simulink model "test_dram_vacc_out"  (Simulink 6.2)
settings: Solver=ode45  StartTime=0.0  StopTime=30000  RelTol=1e-3
undefined symbols (not defined in the file): ant_bits, blockCountBits, blockRowBits
libraries: xbsIndex_r3 x678, xps_library x31, casper_library x10
(part 1 of 4)
settings Model: LastModifiedBy=Jason Manley
settings DebuggingCC: SolverPrmCheckMsg=warning

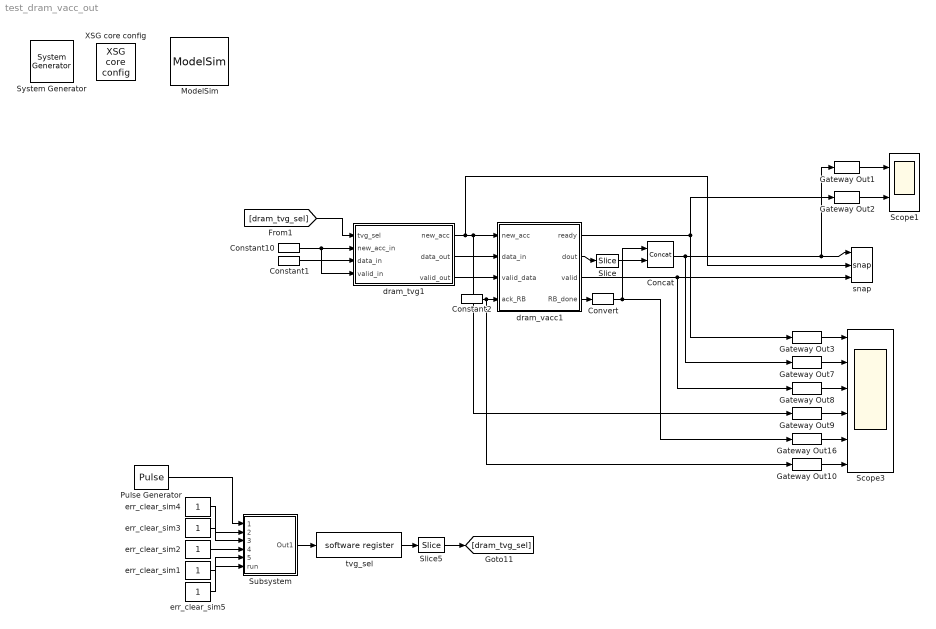
== system test_dram_vacc_out ==
  " System Generator" : xbsIndex_r3/ System Generator  Tag=genX  xilinxfamily=Virtex2P  part=xc2vp70  speed=-7  package=ff1704  synthesis_tool=XST  directory=./dram_acc_test8/sysgen  testbench=off  simulink_period=1  sysclk_period=4.878  incr_netlist=off  trim_vbits=Everywhere in SubSystem  dbl_ovrd=According to Block Masks  core_generation=According to Block Masks  run_coregen=off  deprecated_control=off  eval_field=0
      settings: AttributesFormatString=System\nGenerator
  Concat : xbsIndex_r3/Concat  num_inputs=2  explicit_period=off  period=1  dbl_ovrd=off
  Constant1 : xbsIndex_r3/Constant  const=0  equ=P=C  arith_type=Unsigned  n_bits=128  bin_pt=0  opselect=C  inp2=PCIN>>17  opr=+  inp1=P  carry=CIN  iostate=0  explicit_period=on  period=1  dbl_ovrd=off
  Constant10 : xbsIndex_r3/Constant  const=0  equ=P=C  arith_type=Boolean  n_bits=1  bin_pt=0  opselect=C  inp2=PCIN>>17  opr=+  inp1=P  carry=CIN  iostate=0  explicit_period=on  period=1  dbl_ovrd=off
  Constant2 : xbsIndex_r3/Constant  const=1  equ=P=C  arith_type=Boolean  n_bits=1  bin_pt=0  opselect=C  inp2=PCIN>>17  opr=+  inp1=P  carry=CIN  iostate=0  explicit_period=on  period=1  dbl_ovrd=off
  Convert : xbsIndex_r3/Convert  arith_type=Unsigned  n_bits=1  bin_pt=0  quantization=Truncate  overflow=Wrap  latency=0  explicit_period=off  period=1  dbl_ovrd=off  show_param=off  inserted_by_tool=off  pipeline=off
      settings: xl_area=[0, 0, 0, 0, 0, 0, 0]
  Gateway Out{1..3,7..10,16} (8 alike) : xbsIndex_r3/Gateway Out  output_type=Double  nbits=8  bin_pt=6  arith_type=Boolean  quantization=Truncate  overflow=Wrap  hdl_port=off  timing_constraint=None  locs_specified=off  LOCs={}  needs_fixed_name=off  show_param=off
      settings: xl_area=[0, 0, 0, 0, 0, 0, 0]
  ModelSim : xbsIndex_r3/ModelSim  dir=./modelsim  waveform=on  leave_open=on  skip_compile=off  custom_scripts=off  startup_timeout=40
  Pulse Generator : DiscretePulseGenerator  Period=3000  PhaseDelay=600
  Scope1 : Scope  NumInputPorts=2
      settings: YMin=11.4~0.95  YMax=12.6~1.05
  Scope3 : Scope  NumInputPorts=6
      settings: YMin=0.95~3.8~0~-1~-1~-5  YMax=1.05~4.2~1~1~1~5  SaveName=ScopeData2
  Slice : xbsIndex_r3/Slice  mode=Lower Bit Location + Width  nbits=32  bit1=0  base1=MSB of Input  bit0=0  base0=LSB of Input  boolean_output=off  explicit_period=off  period=1  dbl_ovrd=off
  Slice5 : xbsIndex_r3/Slice  mode=Lower Bit Location + Width  nbits=6  bit1=0  base1=MSB of Input  bit0=9  base0=LSB of Input  boolean_output=off  explicit_period=off  period=1  dbl_ovrd=off
  Subsystem : Subsystem
  XSG core config : xps_library/XSG core config  Tag=xps:xsg  hw_sys=BEE2_usr  ibob_linux=off  clk_src=sys_clk2x  gpio_clk_io_group=iBOB:sma  gpio_clk_bit_index=0  clk_rate=205  sample_period=1  synthesis_tool=XST  mpc_type=powerpc405
  dram_tvg1 : Subsystem  mask{len=100}
      mask prompts: len "Number of Vectors"
      mask init:
      | fmtstr = sprintf('Vector Length: %d', len);
      | set_param(gcb, 'AttributesFormatString', fmtstr);
      settings: AttributesFormatString=Vector Length: 100
  dram_vacc1 : Subsystem  mask{acc_length=100}
      mask prompts: acc_length "Vector length??(# cycles)"
      mask init:
      | valid_length = 36;
  err_clear_sim{1..5} (5 alike) : Constant
  snap : casper_library/Scopes/snap  nsamples=14
  tvg_sel : xps_library/software register  Tag=xps:sw_reg  io_dir=From Processor  arith_type=Unsigned  bitwidth=32  bin_pt=0  sample_period=1  gw_name=test_dram_vacc_out_tvg_sel_user_data_out
  wires:
  Gateway Out1/1 -> Scope1/1
  dram_vacc1/2(dout) -> Slice/1
  dram_vacc1/3(valid) -> Gateway Out8/1, snap/3
  dram_vacc1/4(RB_done) -> Convert/1
  dram_vacc1/1(ready) -> Gateway Out2/1, Gateway Out3/1
  Gateway Out2/1 -> Scope1/2
  Gateway Out3/1 -> Scope3/1
  Gateway Out7/1 -> Scope3/2
  Gateway Out8/1 -> Scope3/3
  Gateway Out9/1 -> Scope3/4
  Gateway Out16/1 -> Scope3/5
  Gateway Out10/1 -> Scope3/6
  tvg_sel/1 -> Slice5/1
  Slice5/1 -> [dram_tvg_sel]
  [dram_tvg_sel] -> dram_tvg1/1(tvg_sel)
  Constant10/1 -> dram_tvg1/4(valid_in), dram_tvg1/2(new_acc_in)
  Constant1/1 -> dram_tvg1/3(data_in)
  err_clear_sim1/1 -> Subsystem/5(data_sel)
  err_clear_sim2/1 -> Subsystem/4(valid_sel)
  err_clear_sim3/1 -> Subsystem/3(inj_vector)
  err_clear_sim4/1 -> Subsystem/2(inj_counter)
  Subsystem/1(Out1) -> tvg_sel/1
  Pulse Generator/1 -> Subsystem/1(new_acc)
  err_clear_sim5/1 -> Subsystem/6(run)
  dram_tvg1/1(new_acc) -> dram_vacc1/1(new_acc), Gateway Out9/1, snap/2
  dram_tvg1/2(data_out) -> dram_vacc1/2(data_in)
  dram_tvg1/3(valid_out) -> dram_vacc1/3(valid_data)
  Constant2/1 -> dram_vacc1/4(ack_RB), Gateway Out10/1
  Concat/1 -> Gateway Out7/1, Gateway Out1/1, snap/1
  Slice/1 -> Concat/2
  Convert/1 -> Gateway Out16/1, Concat/1

== system test_dram_vacc_out/Subsystem ==
  new_acc : Inport  Port=1  LatchInput=off
  inj_counter : Inport  Port=2  LatchInput=off
  inj_vector : Inport  Port=3  LatchInput=off
  valid_sel : Inport  Port=4  LatchInput=off
  data_sel : Inport  Port=5  LatchInput=off
  run : Inport  Port=6  LatchInput=off
  Sum : Sum  Inputs=|++++++
  data_sel1 : Subsystem  mask{bit_pos=10}
      mask prompts: bit_pos "bit position"
  inj_counter1 : Subsystem  mask{bit_pos=13}
      mask prompts: bit_pos "bit position"
  inj_vector1 : Subsystem  mask{bit_pos=12}
      mask prompts: bit_pos "bit position"
  new_acc2 : Subsystem  mask{bit_pos=14}
      mask prompts: bit_pos "bit position"
  run1 : Subsystem  mask{bit_pos=9}
      mask prompts: bit_pos "bit position"
  valid_sel1 : Subsystem  mask{bit_pos=11}
      mask prompts: bit_pos "bit position"
  Out1 : Outport
  wires:
  new_acc2/1(Out1) -> Sum/1
  inj_counter1/1(Out1) -> Sum/2
  inj_vector1/1(Out1) -> Sum/3
  valid_sel1/1(Out1) -> Sum/4
  data_sel1/1(Out1) -> Sum/5
  run1/1(Out1) -> Sum/6
  new_acc/1 -> new_acc2/1(In1)
  inj_counter/1 -> inj_counter1/1(In1)
  inj_vector/1 -> inj_vector1/1(In1)
  valid_sel/1 -> valid_sel1/1(In1)
  Sum/1 -> Out1/1
  data_sel/1 -> data_sel1/1(In1)
  run/1 -> run1/1(In1)

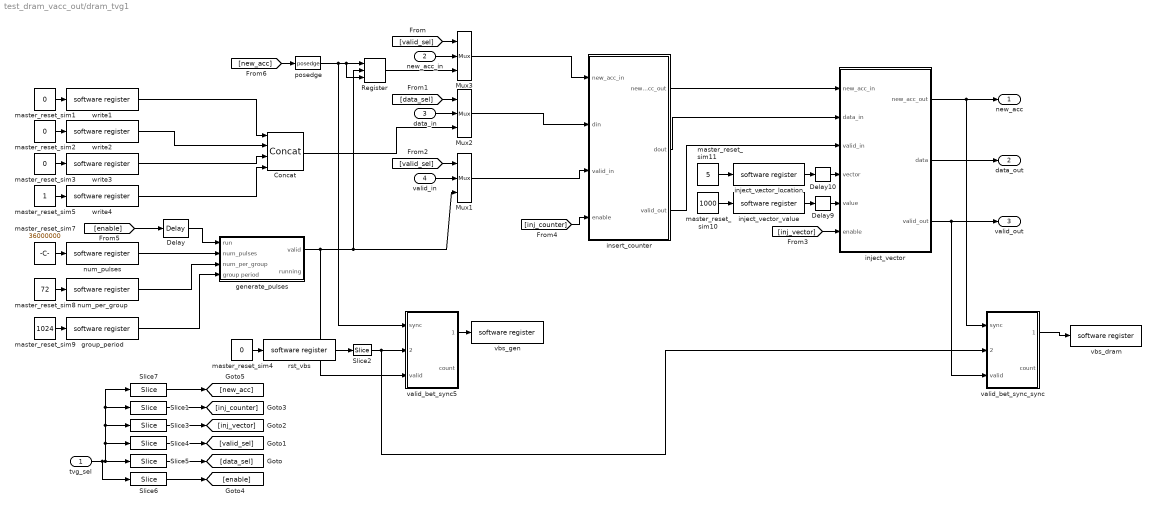
== system test_dram_vacc_out/dram_tvg1 ==
  tvg_sel : Inport  Port=1  LatchInput=off
  new_acc_in : Inport  Port=2  LatchInput=off
  data_in : Inport  Port=3  LatchInput=off
  valid_in : Inport  Port=4  LatchInput=off
  Concat : xbsIndex_r3/Concat  num_inputs=4  explicit_period=on  period=1  dbl_ovrd=off
  Delay : xbsIndex_r3/Delay  latency=1  reg_retiming=on  explicit_period=off  period=1  en=off  accept_only_valid=off  init_zero=on  dbl_ovrd=off  show_param=off
      settings: xl_area=[0, 0, 0, 0, 0, 0, 0]
  Delay10 : xbsIndex_r3/Delay  latency=5  reg_retiming=off  explicit_period=off  period=1  en=off  accept_only_valid=off  init_zero=on  dbl_ovrd=off  show_param=off
      settings: xl_area=[0, 0, 0, 0, 0, 0, 0]
  Delay9 : xbsIndex_r3/Delay  latency=5  reg_retiming=off  explicit_period=off  period=1  en=off  accept_only_valid=off  init_zero=on  dbl_ovrd=off  show_param=off
      settings: xl_area=[0, 0, 0, 0, 0, 0, 0]
  Mux1 : xbsIndex_r3/Mux  inputs=2  precision=Full  arith_type="Signed  (2's comp)"  n_bits=8  bin_pt=2  quantization=Truncate  overflow=Wrap  latency=0  explicit_period=off  period=1  en=off  dbl_ovrd=off  show_param=off  mux_type=off  use_rpm=off  gen_core=off
      settings: xl_area=[0, 0, 0, 0, 0, 0, 0]
  Mux2 : xbsIndex_r3/Mux  inputs=2  precision=Full  arith_type="Signed  (2's comp)"  n_bits=8  bin_pt=2  quantization=Truncate  overflow=Wrap  latency=0  explicit_period=off  period=1  en=off  dbl_ovrd=off  show_param=off  mux_type=off  use_rpm=off  gen_core=off
      settings: xl_area=[0, 0, 0, 0, 0, 0, 0]
  Mux3 : xbsIndex_r3/Mux  inputs=2  precision=Full  arith_type="Signed  (2's comp)"  n_bits=8  bin_pt=2  quantization=Truncate  overflow=Wrap  latency=0  explicit_period=off  period=1  en=off  dbl_ovrd=off  show_param=off  mux_type=off  use_rpm=off  gen_core=off
      settings: xl_area=[0, 0, 0, 0, 0, 0, 0]
  Register : xbsIndex_r3/Register  init=0  reg_only_valid=off  explicit_period=off  period=1  rst=on  en=on  out_en=off  dbl_ovrd=off  show_param=off
      settings: xl_area=[0, 0, 0, 0, 0, 0, 0]
  Slice1 : xbsIndex_r3/Slice  mode=Lower Bit Location + Width  nbits=1  bit1=0  base1=MSB of Input  bit0=4  base0=LSB of Input  boolean_output=on  explicit_period=off  period=1  dbl_ovrd=off
  Slice2 : xbsIndex_r3/Slice  mode=Lower Bit Location + Width  nbits=1  bit1=0  base1=MSB of Input  bit0=0  base0=LSB of Input  boolean_output=on  explicit_period=off  period=1  dbl_ovrd=off
  Slice3 : xbsIndex_r3/Slice  mode=Lower Bit Location + Width  nbits=1  bit1=0  base1=MSB of Input  bit0=3  base0=LSB of Input  boolean_output=on  explicit_period=off  period=1  dbl_ovrd=off
  Slice4 : xbsIndex_r3/Slice  mode=Lower Bit Location + Width  nbits=1  bit1=0  base1=MSB of Input  bit0=2  base0=LSB of Input  boolean_output=on  explicit_period=off  period=1  dbl_ovrd=off
  Slice5 : xbsIndex_r3/Slice  mode=Lower Bit Location + Width  nbits=1  bit1=0  base1=MSB of Input  bit0=1  base0=LSB of Input  boolean_output=on  explicit_period=off  period=1  dbl_ovrd=off
  Slice6 : xbsIndex_r3/Slice  mode=Lower Bit Location + Width  nbits=1  bit1=0  base1=MSB of Input  bit0=0  base0=LSB of Input  boolean_output=on  explicit_period=off  period=1  dbl_ovrd=off
  Slice7 : xbsIndex_r3/Slice  mode=Lower Bit Location + Width  nbits=1  bit1=0  base1=MSB of Input  bit0=5  base0=LSB of Input  boolean_output=on  explicit_period=off  period=1  dbl_ovrd=off
  generate_pulses : Subsystem
  group_period : xps_library/software register  Tag=xps:sw_reg  io_dir=From Processor  arith_type=Unsigned  bitwidth=32  bin_pt=0  sample_period=1  gw_name=test_dram_vacc_out_dram_tvg1_group_period_user_data_out
  inject_vector : Subsystem  mask{num_vectors=len}
      mask prompts: num_vectors "number of vectors"
      mask init:
      | fmtstr = sprintf('Vector Length: %d', num_vectors);
      | set_param(gcb, 'AttributesFormatString', fmtstr);
      settings: AttributesFormatString=Vector Length: 18432
  inject_vector_location : xps_library/software register  Tag=xps:sw_reg  io_dir=From Processor  arith_type=Unsigned  bitwidth=32  bin_pt=0  sample_period=1  gw_name=test_dram_vacc_out_dram_tvg1_inject_vector_location_user_data_out
  inject_vector_value : xps_library/software register  Tag=xps:sw_reg  io_dir=From Processor  arith_type=Unsigned  bitwidth=32  bin_pt=0  sample_period=1  gw_name=test_dram_vacc_out_dram_tvg1_inject_vector_value_user_data_out
  insert_counter : Subsystem  mask{vec_len=len}
      mask prompts: vec_len "Vector Length?"
      mask init:
      | fmtstr = sprintf('Vector Length: %d', vec_len);
      | set_param(gcb, 'AttributesFormatString', fmtstr);
      settings: AttributesFormatString=Vector Length: 18432
  master_reset_sim{1..4} (4 alike) : Constant  Value=0
  master_reset_sim10 : Constant  Value=1000
  master_reset_sim11 : Constant  Value=5
  master_reset_sim5 : Constant
  master_reset_sim7 : Constant  Value=36000000
  master_reset_sim8 : Constant  Value=72
  master_reset_sim9 : Constant  Value=1024
  num_per_group : xps_library/software register  Tag=xps:sw_reg  io_dir=From Processor  arith_type=Unsigned  bitwidth=32  bin_pt=0  sample_period=1  gw_name=test_dram_vacc_out_dram_tvg1_num_per_group_user_data_out
  num_pulses : xps_library/software register  Tag=xps:sw_reg  io_dir=From Processor  arith_type=Unsigned  bitwidth=32  bin_pt=0  sample_period=1  gw_name=test_dram_vacc_out_dram_tvg1_num_pulses_user_data_out
  posedge : casper_library/Misc/posedge  Tag=Rising Edge Detector
  rst_vbs : xps_library/software register  Tag=xps:sw_reg  io_dir=From Processor  arith_type=Unsigned  bitwidth=32  bin_pt=0  sample_period=1  gw_name=test_dram_vacc_out_dram_tvg1_rst_vbs_user_data_out
  valid_bet_sync5 : Subsystem
  valid_bet_sync_sync : Subsystem
  vbs_dram : xps_library/software register  Tag=xps:sw_reg  io_dir=To Processor  arith_type=Unsigned  bitwidth=32  bin_pt=0  sample_period=1  gw_name=test_dram_vacc_out_dram_tvg1_vbs_dram_user_data_in
  vbs_gen : xps_library/software register  Tag=xps:sw_reg  io_dir=To Processor  arith_type=Unsigned  bitwidth=32  bin_pt=0  sample_period=1  gw_name=test_dram_vacc_out_dram_tvg1_vbs_gen_user_data_in
  write1 : xps_library/software register  Tag=xps:sw_reg  io_dir=From Processor  arith_type=Unsigned  bitwidth=32  bin_pt=0  sample_period=1  gw_name=test_dram_vacc_out_dram_tvg1_write1_user_data_out
  write2 : xps_library/software register  Tag=xps:sw_reg  io_dir=From Processor  arith_type=Unsigned  bitwidth=32  bin_pt=0  sample_period=1  gw_name=test_dram_vacc_out_dram_tvg1_write2_user_data_out
  write3 : xps_library/software register  Tag=xps:sw_reg  io_dir=From Processor  arith_type=Unsigned  bitwidth=32  bin_pt=0  sample_period=1  gw_name=test_dram_vacc_out_dram_tvg1_write3_user_data_out
  write4 : xps_library/software register  Tag=xps:sw_reg  io_dir=From Processor  arith_type=Unsigned  bitwidth=32  bin_pt=0  sample_period=1  gw_name=test_dram_vacc_out_dram_tvg1_write4_user_data_out
  new_acc : Outport
  data_out : Outport  Port=2
  valid_out : Outport  Port=3
  wires:
  write1/1 -> Concat/1
  master_reset_sim1/1 -> write1/1
  write2/1 -> Concat/2
  master_reset_sim2/1 -> write2/1
  write3/1 -> Concat/3
  master_reset_sim3/1 -> write3/1
  write4/1 -> Concat/4
  master_reset_sim5/1 -> write4/1
  [new_acc] -> posedge/1
  num_pulses/1 -> generate_pulses/2(num_pulses)
  master_reset_sim7/1 -> num_pulses/1
  num_per_group/1 -> generate_pulses/3(num_per_group)
  master_reset_sim8/1 -> num_per_group/1
  group_period/1 -> generate_pulses/4(group period)
  master_reset_sim9/1 -> group_period/1
  Mux1/1 -> insert_counter/3(valid_in)
  valid_in/1 -> Mux1/2
  inject_vector/1(new_acc_out) -> new_acc/1, valid_bet_sync_sync/1(sync)
  inject_vector/2(data) -> data_out/1
  inject_vector/3(valid_out) -> valid_out/1, valid_bet_sync_sync/3(valid)
  insert_counter/1(new_acc_out) -> inject_vector/1(new_acc_in)
  Mux2/1 -> insert_counter/2(din)
  data_in/1 -> Mux2/2
  new_acc_in/1 -> Mux3/2
  Mux3/1 -> insert_counter/1(new_acc_in)
  Slice5/1 -> [data_sel]
  tvg_sel/1 -> Slice5/1, Slice3/1, Slice1/1, Slice7/1, Slice4/1, Slice6/1
  Slice4/1 -> [valid_sel]
  [valid_sel] -> Mux3/1
  [data_sel] -> Mux2/1
  [valid_sel] -> Mux1/1
  Slice3/1 -> [inj_vector]
  Slice1/1 -> [inj_counter]
  [enable] -> Delay/1
  insert_counter/2(dout) -> inject_vector/2(data_in)
  insert_counter/3(valid_out) -> inject_vector/3(valid_in)
  Concat/1 -> Mux2/3
  generate_pulses/1(valid) -> Register/2, Mux1/3, valid_bet_sync5/3(valid)
  Register/1 -> Mux3/3
  posedge/1 -> Register/1, Register/3, valid_bet_sync5/1(sync)
  [inj_vector] -> inject_vector/6(enable)
  Delay10/1 -> inject_vector/4(vector)
  master_reset_sim11/1 -> inject_vector_location/1
  inject_vector_location/1 -> Delay10/1
  Delay9/1 -> inject_vector/5(value)
  master_reset_sim10/1 -> inject_vector_value/1
  inject_vector_value/1 -> Delay9/1
  [inj_counter] -> insert_counter/4(enable)
  Slice6/1 -> [enable]
  Slice7/1 -> [new_acc]
  valid_bet_sync5/1(max_count) -> vbs_gen/1
  master_reset_sim4/1 -> rst_vbs/1
  Slice2/1 -> valid_bet_sync5/2(rst_max), valid_bet_sync_sync/2(rst_max)
  rst_vbs/1 -> Slice2/1
  valid_bet_sync_sync/1(max_count) -> vbs_dram/1
  Delay/1 -> generate_pulses/1(run)

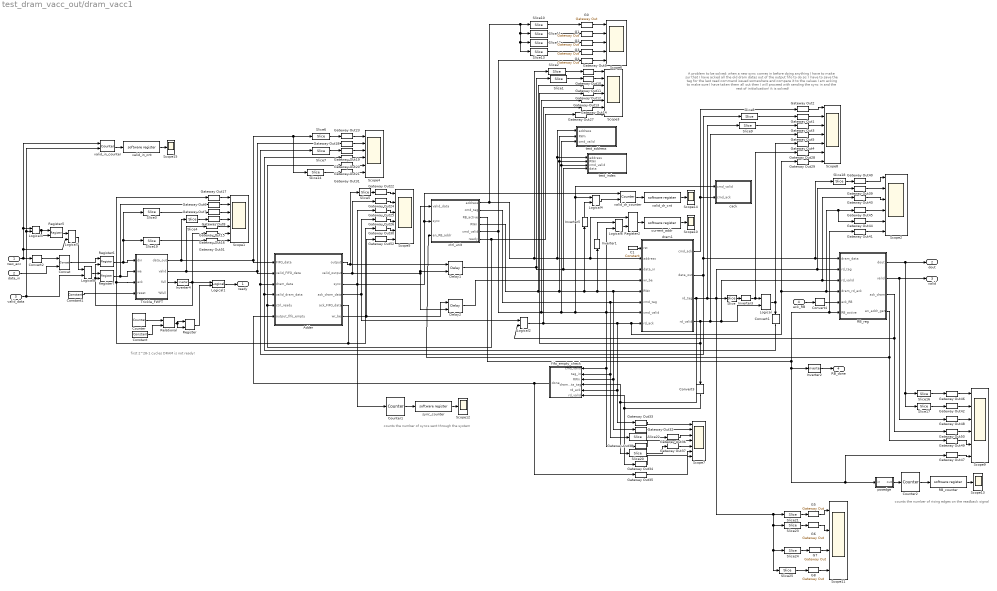
== system test_dram_vacc_out/dram_vacc1 ==
  note: counts the number of rising edges on
      | the readback signal
  note: counts the number of syncs
      | sent through the system
  note: first 2^28-1 cycles DRAM
      | is not ready!
  note: A problem to be solved:
      | when a new sync comes in before doing anything I have to make sur
      | that I have acked all the old dram datas out of the output fifo
      | to do so: I have to save the tag for the last read command issued somewhere
      | and compare it to the values I am acking to make sure I have taken them all out
      | then I will proceed with sending the sync in and the rest of initialization!
      | it is solved!
  new_acc : Inport  Port=1  LatchInput=off
  data_in : Inport  Port=2  LatchInput=off
  valid_data : Inport  Port=3  LatchInput=off
  ack_RB : Inport  Port=4  LatchInput=off
  Adder : Subsystem
  C1 : xbsIndex_r3/Constant  const=0  equ=P=C  arith_type=Boolean  n_bits=1  bin_pt=0  opselect=C  inp2=PCIN>>17  opr=+  inp1=P  carry=CIN  iostate=0  explicit_period=on  period=1  dbl_ovrd=off
  Concat : xbsIndex_r3/Concat  num_inputs=2  explicit_period=off  period=1  dbl_ovrd=off
  Constant : xbsIndex_r3/Constant  const=2^28-1  equ=P=C  arith_type=Unsigned  n_bits=28  bin_pt=0  opselect=C  inp2=PCIN>>17  opr=+  inp1=P  carry=CIN  iostate=0  explicit_period=on  period=1  dbl_ovrd=off
  Constant1 : xbsIndex_r3/Constant  const=0  equ=P=C  arith_type=Boolean  n_bits=28  bin_pt=0  opselect=C  inp2=PCIN>>17  opr=+  inp1=P  carry=CIN  iostate=0  explicit_period=on  period=1  dbl_ovrd=off
  Convert1 : xbsIndex_r3/Convert  Orientation=down  arith_type=Boolean  n_bits=31  bin_pt=0  quantization=Truncate  overflow=Wrap  latency=0  explicit_period=off  period=1  dbl_ovrd=off  show_param=off  inserted_by_tool=off  pipeline=off
      settings: xl_area=[0, 0, 0, 0, 0, 0, 0]
  Convert2 : xbsIndex_r3/Convert  arith_type=Unsigned  n_bits=1  bin_pt=0  quantization=Truncate  overflow=Wrap  latency=0  explicit_period=off  period=1  dbl_ovrd=off  show_param=off  inserted_by_tool=off  pipeline=off
      settings: xl_area=[0, 0, 0, 0, 0, 0, 0]
  Convert3 : xbsIndex_r3/Convert  Orientation=down  arith_type=Boolean  n_bits=31  bin_pt=0  quantization=Truncate  overflow=Wrap  latency=0  explicit_period=off  period=1  dbl_ovrd=off  show_param=off  inserted_by_tool=off  pipeline=off
      settings: xl_area=[0, 0, 0, 0, 0, 0, 0]
  Convert4 : xbsIndex_r3/Convert  arith_type=Boolean  n_bits=31  bin_pt=0  quantization=Truncate  overflow=Wrap  latency=0  explicit_period=off  period=1  dbl_ovrd=off  show_param=off  inserted_by_tool=off  pipeline=off
      settings: xl_area=[0, 0, 0, 0, 0, 0, 0]
  Counter : xbsIndex_r3/Counter  cnt_type=Free Running  n_bits=28  bin_pt=0  arith_type=Unsigned  start_count=0  cnt_to=Inf  cnt_by_val=1  operation=Up  explicit_period=off  period=1  load_pin=off  rst=off  en=off  dbl_ovrd=off  show_param=off  use_rpm=on  gen_core=off
      settings: xl_area=[0, 0, 0, 0, 0, 0, 0]
  Counter1 : xbsIndex_r3/Counter  cnt_type=Free Running  n_bits=10  bin_pt=0  arith_type=Unsigned  start_count=0  cnt_to=Inf  cnt_by_val=1  operation=Up  explicit_period=off  period=1  load_pin=off  rst=off  en=on  dbl_ovrd=off  show_param=off  use_rpm=on  gen_core=off
      settings: xl_area=[0, 0, 0, 0, 0, 0, 0]
  Counter2 : xbsIndex_r3/Counter  cnt_type=Free Running  n_bits=10  bin_pt=0  arith_type=Unsigned  start_count=0  cnt_to=Inf  cnt_by_val=1  operation=Up  explicit_period=off  period=1  load_pin=off  rst=off  en=on  dbl_ovrd=off  show_param=off  use_rpm=on  gen_core=off
      settings: xl_area=[0, 0, 0, 0, 0, 0, 0]
  Delay1 : xbsIndex_r3/Delay  latency=1  reg_retiming=off  explicit_period=on  period=1  en=on  accept_only_valid=off  init_zero=on  dbl_ovrd=off  show_param=off
      settings: xl_area=[0, 0, 0, 0, 0, 0, 0]
  Delay2 : xbsIndex_r3/Delay  latency=1  reg_retiming=off  explicit_period=on  period=1  en=on  accept_only_valid=off  init_zero=on  dbl_ovrd=off  show_param=off
      settings: xl_area=[0, 0, 0, 0, 0, 0, 0]
  G{0..8} (9 alike) : xbsIndex_r3/Gateway Out  output_type=Double  nbits=8  bin_pt=6  arith_type=Boolean  quantization=Truncate  overflow=Wrap  hdl_port=off  timing_constraint=None  locs_specified=off  LOCs={}  needs_fixed_name=off  show_param=off
      settings: xl_area=[0, 0, 0, 0, 0, 0, 0]
  Gateway Out{1..52} (52 alike) : xbsIndex_r3/Gateway Out  output_type=Double  nbits=8  bin_pt=6  arith_type=Boolean  quantization=Truncate  overflow=Wrap  hdl_port=off  timing_constraint=None  locs_specified=off  LOCs={}  needs_fixed_name=off  show_param=off
      settings: xl_area=[0, 0, 0, 0, 0, 0, 0]
  Inverter1 : xbsIndex_r3/Inverter  Orientation=up  latency=0  explicit_period=off  period=1  en=off  dbl_ovrd=off  show_param=off
      settings: xl_area=[0, 0, 0, 0, 0, 0, 0]
  Inverter2 : xbsIndex_r3/Inverter  latency=0  explicit_period=off  period=1  en=off  dbl_ovrd=off  show_param=off
      settings: xl_area=[0, 0, 0, 0, 0, 0, 0]
  Inverter3 : xbsIndex_r3/Inverter  latency=0  explicit_period=off  period=1  en=off  dbl_ovrd=off  show_param=off
      settings: xl_area=[0, 0, 0, 0, 0, 0, 0]
  Inverter4 : xbsIndex_r3/Inverter  latency=0  explicit_period=off  period=1  en=off  dbl_ovrd=off  show_param=off
      settings: xl_area=[0, 0, 0, 0, 0, 0, 0]
  Inverter5 : xbsIndex_r3/Inverter  Orientation=up  latency=0  explicit_period=off  period=1  en=off  dbl_ovrd=off  show_param=off
      settings: xl_area=[0, 0, 0, 0, 0, 0, 0]
  Logical{,1,3..4,6,8} (6 alike) : xbsIndex_r3/Logical  logical_function=AND  inputs=2  precision=Full  arith_type=Unsigned  n_bits=8  bin_pt=2  align_bp=on  latency=0  explicit_period=off  period=1  en=off  dbl_ovrd=off  show_param=off
      settings: xl_area=[0, 0, 0, 0, 0, 0, 0]
  Logical2 : xbsIndex_r3/Logical  logical_function=OR  inputs=2  precision=Full  arith_type=Unsigned  n_bits=8  bin_pt=2  align_bp=on  latency=0  explicit_period=off  period=1  en=off  dbl_ovrd=off  show_param=off
      settings: xl_area=[0, 0, 0, 0, 0, 0, 0]
  Logical7 : xbsIndex_r3/Logical  logical_function=OR  inputs=2  precision=Full  arith_type=Unsigned  n_bits=8  bin_pt=2  align_bp=on  latency=0  explicit_period=off  period=1  en=off  dbl_ovrd=off  show_param=off
      settings: xl_area=[0, 0, 0, 0, 0, 0, 0]
  RB_counter : xps_library/software register  Tag=xps:sw_reg  io_dir=To Processor  arith_type=Unsigned  bitwidth=32  bin_pt=0  sample_period=1  gw_name=test_dram_vacc_out_dram_vacc1_RB_counter_user_data_in
  RB_reg : Subsystem
  Register{,2,5..7} (5 alike) : xbsIndex_r3/Register  init=0  reg_only_valid=off  explicit_period=off  period=1  rst=off  en=on  out_en=off  dbl_ovrd=off  show_param=off
      settings: xl_area=[0, 0, 0, 0, 0, 0, 0]
  Relational : xbsIndex_r3/Relational  mode=a=b  latency=1  explicit_period=off  period=1  en=off  dbl_ovrd=off  show_param=off
      settings: xl_area=[0, 0, 0, 0, 0, 0, 0]
  Scope{1,3,7..8} (4 alike) : Scope  NumInputPorts=7
      Scope1 settings: TimeRange=30000  YMin=0~0~0.95~0.95~0~0.95~-1  YMax=1~1~1.05~1.05~1~1.05~1  SaveName=ScopeData7
      Scope3 settings: YMin=0~0~0~0~0~0~0  YMax=150~2500~1~1~1~1~1  SaveName=ScopeData6
      Scope7 settings: YMin=0~0~0~0~0~0.95~0  YMax=1~1100~7500~1~1~1.05~1  SaveName=ScopeData17
      Scope8 settings: YMin=0~0~2.68438e+008~0~0~0~0  YMax=1~11000~2.68439e+008~1~1~1~1  SaveName=ScopeData19
  Scope{10,12..15} (5 alike) : Scope
      Scope10 settings: YMin=0  YMax=100  SaveName=ScopeData27
      Scope12 settings: YMin=0  YMax=100  SaveName=ScopeData32
      Scope13 settings: YMin=0  YMax=100  SaveName=ScopeData33
      Scope14 settings: YMin=0  YMax=100  SaveName=ScopeData21
      Scope15 settings: YMin=0  YMax=100  SaveName=ScopeData24
  Scope11 : Scope  NumInputPorts=4
      settings: YMin=0~0.95~-1~1.9  YMax=120~1.05~1~2.1  SaveName=ScopeData28
  Scope{2,4..5,9} (4 alike) : Scope  NumInputPorts=6
      Scope2 settings: YMin=2.5~5e+008~0~0~0~0.95  YMax=12.5~2.75e+009~1~1~1~1.05  SaveName=ScopeData22
      Scope4 settings: YMin=0.95~0.95~-1~-1~0.95~-1  YMax=1.05~1.05~1~1~1.05~1  SaveName=ScopeData8
      Scope5 settings: YMin=0~0~-1~0~0~-5  YMax=250~1~1~1~1~5  SaveName=ScopeData9
      Scope9 settings: YMin=1.9~1.9~-1~0~-1~0.95  YMax=2.1~2.1~1~1~1~1.05  SaveName=ScopeData23
  Scope6 : Scope  NumInputPorts=5
      settings: YMin=0~0~0~0~0  YMax=200~4000~1~1~1  SaveName=ScopeData14
  Slice : xbsIndex_r3/Slice  mode=Upper Bit Location + Width  nbits=1  bit1=0  base1=MSB of Input  bit0=0  base0=LSB of Input  boolean_output=off  explicit_period=off  period=1  dbl_ovrd=off
  Slice{1,3..8,16..18} (10 alike) : xbsIndex_r3/Slice  mode=Lower Bit Location + Width  nbits=32  bit1=0  base1=MSB of Input  bit0=0  base0=LSB of Input  boolean_output=off  explicit_period=off  period=1  dbl_ovrd=off
  Slice{2,10,20,22} (4 alike) : xbsIndex_r3/Slice  mode=Lower Bit Location + Width  nbits=8  bit1=0  base1=MSB of Input  bit0=5  base0=LSB of Input  boolean_output=off  explicit_period=off  period=1  dbl_ovrd=off
  Slice11 : xbsIndex_r3/Slice  mode=Lower Bit Location + Width  nbits=14  bit1=0  base1=MSB of Input  bit0=14  base0=LSB of Input  boolean_output=off  explicit_period=off  period=1  dbl_ovrd=off
  Slice12 : xbsIndex_r3/Slice  mode=Lower Bit Location + Width  nbits=1  bit1=0  base1=MSB of Input  bit0=13  base0=LSB of Input  boolean_output=off  explicit_period=off  period=1  dbl_ovrd=off
  Slice13 : xbsIndex_r3/Slice  mode=Lower Bit Location + Width  nbits=2  bit1=0  base1=MSB of Input  bit0=28  base0=LSB of Input  boolean_output=off  explicit_period=off  period=1  dbl_ovrd=off
  Slice14 : xbsIndex_r3/Slice  mode=Upper Bit Location + Width  nbits=1  bit1=0  base1=MSB of Input  bit0=0  base0=LSB of Input  boolean_output=off  explicit_period=off  period=1  dbl_ovrd=off
  Slice19 : xbsIndex_r3/Slice  mode=Upper Bit Location + Width  nbits=1  bit1=0  base1=MSB of Input  bit0=0  base0=LSB of Input  boolean_output=off  explicit_period=off  period=1  dbl_ovrd=off
  Slice21 : xbsIndex_r3/Slice  mode=Lower Bit Location + Width  nbits=8  bit1=0  base1=MSB of Input  bit0=6  base0=LSB of Input  boolean_output=off  explicit_period=off  period=1  dbl_ovrd=off
  Slice23 : xbsIndex_r3/Slice  mode=Lower Bit Location + Width  nbits=14  bit1=0  base1=MSB of Input  bit0=15  base0=LSB of Input  boolean_output=off  explicit_period=off  period=1  dbl_ovrd=off
  Slice24 : xbsIndex_r3/Slice  mode=Lower Bit Location + Width  nbits=1  bit1=0  base1=MSB of Input  bit0=14  base0=LSB of Input  boolean_output=off  explicit_period=off  period=1  dbl_ovrd=off
  Slice25 : xbsIndex_r3/Slice  mode=Lower Bit Location + Width  nbits=2  bit1=0  base1=MSB of Input  bit0=29  base0=LSB of Input  boolean_output=off  explicit_period=off  period=1  dbl_ovrd=off
  Slice9 : xbsIndex_r3/Slice  mode=Lower Bit Location + Width  nbits=31  bit1=0  base1=MSB of Input  bit0=0  base0=LSB of Input  boolean_output=off  explicit_period=off  period=1  dbl_ovrd=off
  Trickle_FWFT : Subsystem  mask{depth=512}
      mask init:
      | cursys = gcb ; 
      | set_param([cursys, '/FIFO'], 'depth', depth);
      mask StyleString: popup(16|32|64|128|256|512|1K|2K|4K|8K|16K|32K|64K)
  cack : Subsystem
  ctrl_unit : Subsystem  mask{burst_length=valid_length, acc_length=acc_length}
      mask prompts: burst_length "Burst Length?"; acc_length "Accumulation length?"
  current_addr : xps_library/software register  Tag=xps:sw_reg  io_dir=To Processor  arith_type=Unsigned  bitwidth=32  bin_pt=0  sample_period=1  gw_name=test_dram_vacc_out_dram_vacc1_current_addr_user_data_in
  dram1 : Subsystem  Tag=xps:dram  AncestorBlock=xps_library/dram  mask(dram){dimm=1, arith_type=Unsigned, bin_pt=0, ip_clock=200, sample_period=1, use_sim=on, bank_mgt=on, wide_data=off, half_burst=off, shared=on}
      mask prompts: arith_type "Data Type"; bin_pt "Data binary point"; ip_clock "Datapath clock rate (MHz)"; sample_period "Sample period"; use_sim "Simulate DRAM using ModelSim"; bank_mgt "Enable bank management"; wide_data "Use wide data bus (288 bits)"; half_burst "Use half-burst"; shared "Share with PowerPC"
      mask help:
      | Interface to 1GB DDR2 DIMMs on BEE2.
      |
      | To simulate using ModelSim, place a ModelSim block named 'ModelSim' (case-sensitive) in the top level of the design.
      mask init:
      | dram_mask;
      mask StyleString: popup(1|2|3|4),popup(Boolean|Unsigned|Signed  (2's comp)),edit,edit,edit,checkbox,checkbox,checkbox,checkbox,checkbox
      mask CallbackString:
      | |||||||myname=gcb;
      | if strcmp(get_param(myname, 'wide_data'), 'off')
      |     set_param(myname, 'MaskEnables', {'on','on','on','on','on','on','on','on','on','on'});
      | else
      |     set_param(myname, 'half_burst', 'off');
      |     set_param(myname, 'MaskEnables', {'on','on','on','on','on','on','on','on','off','on'});
      | end||
  fifo_empty_check : Subsystem  Orientation=left
  posedge : Subsystem
  sync_counter : xps_library/software register  Tag=xps:sw_reg  io_dir=To Processor  arith_type=Unsigned  bitwidth=32  bin_pt=0  sample_period=1  gw_name=test_dram_vacc_out_dram_vacc1_sync_counter_user_data_in
  test_address : Subsystem
  test_index : Subsystem
  valid_dr_cnt : xps_library/software register  Tag=xps:sw_reg  io_dir=To Processor  arith_type=Unsigned  bitwidth=32  bin_pt=0  sample_period=1  gw_name=test_dram_vacc_out_dram_vacc1_valid_dr_cnt_user_data_in
  valid_dr_counter : xbsIndex_r3/Counter  cnt_type=Count Limited  n_bits=32  bin_pt=0  arith_type=Unsigned  start_count=0  cnt_to=Inf  cnt_by_val=1  operation=Up  explicit_period=off  period=1  load_pin=off  rst=on  en=on  dbl_ovrd=off  show_param=off  use_rpm=on  gen_core=off
      settings: xl_area=[0, 0, 0, 0, 0, 0, 0]
  valid_in_cnt : xps_library/software register  Tag=xps:sw_reg  io_dir=To Processor  arith_type=Unsigned  bitwidth=32  bin_pt=0  sample_period=1  gw_name=test_dram_vacc_out_dram_vacc1_valid_in_cnt_user_data_in
  valid_in_counter : xbsIndex_r3/Counter  cnt_type=Count Limited  n_bits=32  bin_pt=0  arith_type=Unsigned  start_count=0  cnt_to=Inf  cnt_by_val=1  operation=Up  explicit_period=off  period=1  load_pin=off  rst=on  en=on  dbl_ovrd=off  show_param=off  use_rpm=on  gen_core=off
      settings: xl_area=[0, 0, 0, 0, 0, 0, 0]
  ready : Outport
  dout : Outport  Port=2
  valid : Outport  Port=3
  RB_done : Outport  Port=4
  wires:
  Convert4/1 -> RB_reg/5(ack_RB)
  Inverter3/1 -> Gateway Out28/1, Logical/1
  ack_RB/1 -> Convert4/1
  ctrl_unit/5(cmd_valid) -> G4/1, Gateway Out13/1, Logical6/2, Gateway Out38/1, fifo_empty_check/1(cmd_valid), dram1/7(cmd_valid), cack/1(cmd_valid), Logical4/1, test_address/3(cmd_valid), test_index/3(cmd_valid)
  Inverter2/1 -> RB_done/1
  posedge/1(out) -> Counter2/1
  RB_counter/1 -> Scope13/1
  Counter2/1 -> RB_counter/1
  sync_counter/1 -> Scope12/1
  Counter1/1 -> sync_counter/1
  Inverter4/1 -> Logical1/1, Gateway Out16/1, Register7/2, Register6/2
  G8/1 -> Scope11/4
  G7/1 -> Scope11/3
  G6/1 -> Scope11/2
  G5/1 -> Scope11/1
  Slice25/1 -> G8/1
  Slice24/1 -> G7/1
  Slice23/1 -> G6/1
  Slice21/1 -> G5/1
  Slice20/1 -> Gateway Out37/1
  Slice22/1 -> Gateway Out36/1
  current_addr/1 -> Scope10/1
  Inverter1/1 -> Logical6/1
  Logical6/1 -> Register2/2
  Register2/1 -> current_addr/1
  Slice19/1 -> Gateway Out51/1
  Gateway Out51/1 -> Scope1/7
  Register7/1 -> Gateway Out6/1, Trickle_FWFT/2(we)
  Register/1 -> Logical1/2
  Relational/1 -> Register/2, Register/1
  Constant/1 -> Relational/2
  Counter/1 -> Relational/1
  Logical1/1 -> ready/1
  Gateway Out47/1 -> Scope9/6
  Slice18/1 -> Gateway Out40/1
  Slice17/1 -> Gateway Out42/1
  Slice16/1 -> Gateway Out46/1
  Convert3/1 -> Gateway Out34/1, fifo_empty_check/6(rd_valid)
  Gateway Out49/1 -> Scope9/5
  Gateway Out50/1 -> Scope9/4
  Gateway Out48/1 -> Scope9/3
  Gateway Out42/1 -> Scope9/2
  Gateway Out46/1 -> Scope9/1
  Gateway Out41/1 -> Scope2/6
  Gateway Out44/1 -> Scope2/5
  Gateway Out45/1 -> Scope2/4
  Gateway Out43/1 -> Scope2/3
  Gateway Out39/1 -> Scope2/2
  Gateway Out40/1 -> Scope2/1
  Logical2/1 -> Gateway Out14/1, Gateway Out44/1, Gateway Out45/1, RB_reg/4(dram_rd_ack), Gateway Out29/1, dram1/8(rd_ack), Gateway Out33/1, fifo_empty_check/5(rd_ack)
  ctrl_unit/3(RB_active) -> Inverter2/1, posedge/1(in), Gateway Out47/1, RB_reg/6(RB_active), Gateway Out41/1
  RB_reg/4(en_addr_gen) -> Gateway Out49/1, ctrl_unit/3(en_RB_addr)
  RB_reg/3(ack_dram) -> Logical2/2, Gateway Out50/1
  RB_reg/2(valid) -> valid/1, Gateway Out48/1
  RB_reg/1(dout) -> Slice17/1, Slice16/1, dout/1
  Gateway Out29/1 -> Scope8/7
  Gateway Out28/1 -> Scope8/6
  Gateway Out4/1 -> Scope8/5
  Gateway Out5/1 -> Scope8/4
  Gateway Out3/1 -> Scope8/3
  Gateway Out1/1 -> Scope8/2
  Gateway Out2/1 -> Scope8/1
  Gateway Out35/1 -> Scope7/7
  Gateway Out34/1 -> Scope7/6
  Gateway Out38/1 -> Scope7/4
  Gateway Out37/1 -> Scope7/5
  Gateway Out36/1 -> Scope7/3
  Gateway Out32/1 -> Scope7/2
  Gateway Out33/1 -> Scope7/1
  fifo_empty_check/1(done) -> Gateway Out35/1, Adder/6(output_fifo_empty)
  Delay1/1 -> Slice1/1, dram1/3(data_in), test_index/4(data)
  Slice14/1 -> Gateway Out31/1
  Gateway Out31/1 -> Scope4/6
  G4/1 -> Scope6/5
  G3/1 -> Scope6/4
  G2/1 -> Scope6/3
  G1/1 -> Scope6/2
  G0/1 -> Scope6/1
  Slice13/1 -> G3/1
  Slice12/1 -> G2/1
  Slice11/1 -> G1/1
  Slice10/1 -> G0/1
  Gateway Out30/1 -> Scope5/5
  Adder/5(ack_FIFO_data) -> Gateway Out30/1, Gateway Out17/1, Trickle_FWFT/3(ack)
  Slice9/1 -> Gateway Out3/1
  Slice8/1 -> Gateway Out1/1
  Gateway Out27/1 -> Scope3/7
  Slice7/1 -> Gateway Out19/1
  Slice6/1 -> Gateway Out23/1
  Slice5/1 -> Gateway Out22/1
  Convert1/1 -> Adder/4(valid_dram_data), Gateway Out20/1
  Slice4/1 -> Gateway Out8/1
  Slice3/1 -> Gateway Out7/1
  Gateway Out26/1 -> Scope5/4
  Gateway Out25/1 -> Scope5/3
  Gateway Out24/1 -> Scope5/2
  Gateway Out22/1 -> Scope5/1
  Gateway Out21/1 -> Scope4/5
  Gateway Out20/1 -> Scope4/4
  Gateway Out19/1 -> Scope4/3
  Gateway Out18/1 -> Scope4/2
  Gateway Out23/1 -> Scope4/1
  Gateway Out16/1 -> Scope1/6
  Gateway Out15/1 -> Scope1/5
  Gateway Out8/1 -> Scope1/4
  Gateway Out7/1 -> Scope1/3
  Gateway Out6/1 -> Scope1/2
  Gateway Out17/1 -> Scope1/1
  Slice2/1 -> Gateway Out9/1
  Slice1/1 -> Gateway Out10/1
  Gateway Out14/1 -> Scope3/6
  Gateway Out13/1 -> Scope3/5
  Gateway Out12/1 -> Scope3/4
  Gateway Out11/1 -> Scope3/3
  Gateway Out10/1 -> Scope3/2
  Gateway Out9/1 -> Scope3/1
  Register6/1 -> Slice19/1, Slice3/1, Trickle_FWFT/1(din)
  Trickle_FWFT/3(full) -> Inverter4/1
  ctrl_unit/2(cmd_tag) -> Slice22/1, fifo_empty_check/2(tag_in), dram1/6(cmd_tag)
  dram1/1(cmd_ack) -> Gateway Out2/1, cack/2(cmd_ack)
  Adder/3(sync) -> Counter1/1, ctrl_unit/2(sync), valid_dr_counter/1, Gateway Out25/1
  Adder/2(valid_output) -> Gateway Out24/1, Delay1/2, ctrl_unit/1(valid_data), Delay2/2
  ctrl_unit/6(ready) -> Gateway Out27/1, Adder/5(ctrl_ready), Gateway Out21/1
  Logical/1 -> Convert1/1, Gateway Out4/1
  dram1/4(rd_valid) -> Convert3/1, Gateway Out12/1, RB_reg/3(rd_valid), Gateway Out43/1, Logical/2, Gateway Out5/1
  Slice/1 -> Inverter3/1
  dram1/3(rd_tag) -> Slice20/1, fifo_empty_check/4(dram_data_tag), RB_reg/2(rd_tag), Gateway Out39/1, Slice/1, Slice24/1, Slice25/1, Slice23/1, Slice21/1, Slice9/1
  dram1/2(data_out) -> RB_reg/1(dram_data), Slice18/1, Slice8/1, Adder/3(dram_data), Slice7/1
  Adder/1(output) -> Delay1/1, Slice5/1
  C1/1 -> dram1/1(rst)
  ctrl_unit/4(RWn) -> Gateway Out11/1, Inverter1/1, Gateway Out32/1, fifo_empty_check/3(RWn), dram1/5(RWn), Inverter5/1, test_address/2(RWn), test_index/2(RWn)
  ctrl_unit/1(address) -> Slice2/1, Register2/1, dram1/2(address), test_address/1(address), test_index/1(address), Slice12/1, Slice13/1, Slice11/1, Slice10/1
  Trickle_FWFT/2(valid) -> Adder/2(valid_FIFO_data), Gateway Out18/1, Gateway Out15/1
  Trickle_FWFT/1(data_out) -> Slice4/1, Slice14/1, Slice6/1, Adder/1(FIFO_data)
  Adder/4(ack_dram_data) -> Logical2/1, Gateway Out26/1
  new_acc/1 -> Convert2/1, Logical7/2, Logical3/1, valid_in_counter/1
  data_in/1 -> Concat/2
  valid_data/1 -> Logical8/2, Logical3/2, valid_in_counter/2
  Convert2/1 -> Concat/1
  Register5/1 -> Logical7/1
  Logical7/1 -> Logical8/1
  Logical3/1 -> Register5/1, Register5/2
  Concat/1 -> Register6/1
  Logical8/1 -> Register7/1
  Constant1/1 -> Trickle_FWFT/4(reset)
  Logical4/1 -> valid_dr_counter/2
  valid_dr_cnt/1 -> Scope14/1
  valid_dr_counter/1 -> valid_dr_cnt/1
  Inverter5/1 -> Logical4/2
  valid_in_cnt/1 -> Scope15/1
  valid_in_counter/1 -> valid_in_cnt/1
  Adder/6(wr_be) -> Delay2/1, Gateway Out52/1
  Delay2/1 -> dram1/4(wr_be)
  Gateway Out52/1 -> Scope5/6

== system test_dram_vacc_out/Subsystem/data_sel1 ==
  In1 : Inport  Port=1  LatchInput=off
  Product : Product  RndMeth=Zero
  err_clear_sim1 : Constant  Value=2^bit_pos
  Out1 : Outport
  wires:
  err_clear_sim1/1 -> Product/2
  In1/1 -> Product/1
  Product/1 -> Out1/1

== system test_dram_vacc_out/Subsystem/inj_counter1 ==
  In1 : Inport  Port=1  LatchInput=off
  Product : Product  RndMeth=Zero
  err_clear_sim1 : Constant  Value=2^bit_pos
  Out1 : Outport
  wires:
  err_clear_sim1/1 -> Product/2
  In1/1 -> Product/1
  Product/1 -> Out1/1

== system test_dram_vacc_out/Subsystem/inj_vector1 ==
  In1 : Inport  Port=1  LatchInput=off
  Product : Product  RndMeth=Zero
  err_clear_sim1 : Constant  Value=2^bit_pos
  Out1 : Outport
  wires:
  err_clear_sim1/1 -> Product/2
  In1/1 -> Product/1
  Product/1 -> Out1/1

== system test_dram_vacc_out/Subsystem/new_acc2 ==
  In1 : Inport  Port=1  LatchInput=off
  Product : Product  RndMeth=Zero
  err_clear_sim1 : Constant  Value=2^bit_pos
  Out1 : Outport
  wires:
  err_clear_sim1/1 -> Product/2
  In1/1 -> Product/1
  Product/1 -> Out1/1

== system test_dram_vacc_out/Subsystem/run1 ==
  In1 : Inport  Port=1  LatchInput=off
  Product : Product  RndMeth=Zero
  err_clear_sim1 : Constant  Value=2^bit_pos
  Out1 : Outport
  wires:
  err_clear_sim1/1 -> Product/2
  In1/1 -> Product/1
  Product/1 -> Out1/1

== system test_dram_vacc_out/Subsystem/valid_sel1 ==
  In1 : Inport  Port=1  LatchInput=off
  Product : Product  RndMeth=Zero
  err_clear_sim1 : Constant  Value=2^bit_pos
  Out1 : Outport
  wires:
  err_clear_sim1/1 -> Product/2
  In1/1 -> Product/1
  Product/1 -> Out1/1

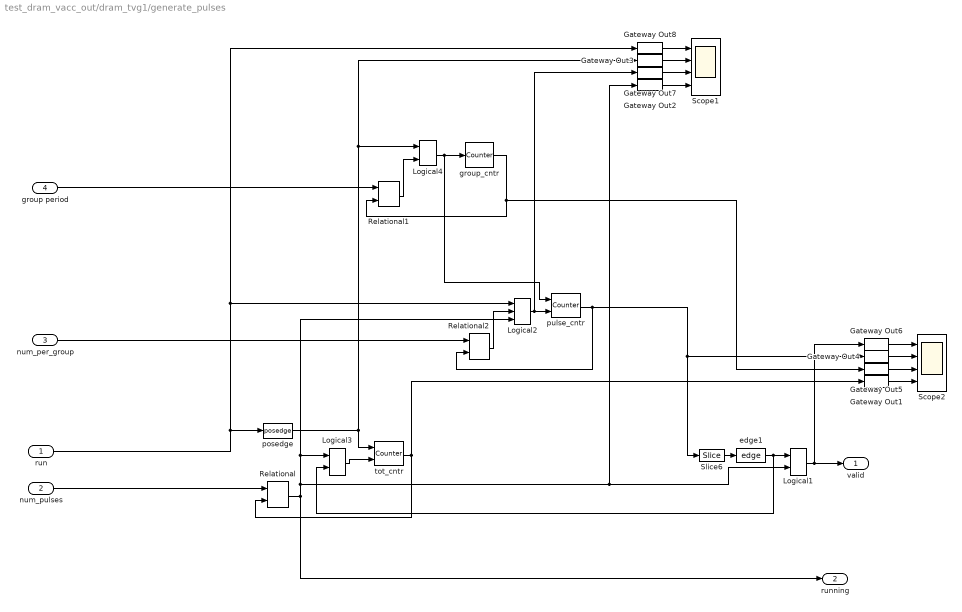
== system test_dram_vacc_out/dram_tvg1/generate_pulses ==
  run : Inport  Port=1  LatchInput=off
  num_pulses : Inport  Port=2  LatchInput=off
  num_per_group : Inport  Port=3  LatchInput=off
  group period : Inport  Port=4  LatchInput=off
  Gateway Out{1..8} (8 alike) : xbsIndex_r3/Gateway Out  output_type=Double  nbits=8  bin_pt=6  arith_type=Boolean  quantization=Truncate  overflow=Wrap  hdl_port=off  timing_constraint=None  locs_specified=off  LOCs={}  needs_fixed_name=off  show_param=off
      settings: xl_area=[0, 0, 0, 0, 0, 0, 0]
  Logical1 : xbsIndex_r3/Logical  logical_function=AND  inputs=2  precision=Full  arith_type=Unsigned  n_bits=8  bin_pt=2  align_bp=on  latency=0  explicit_period=off  period=1  en=off  dbl_ovrd=off  show_param=off
      settings: xl_area=[0, 0, 0, 0, 0, 0, 0]
  Logical2 : xbsIndex_r3/Logical  logical_function=AND  inputs=3  precision=Full  arith_type=Unsigned  n_bits=8  bin_pt=2  align_bp=on  latency=0  explicit_period=off  period=1  en=off  dbl_ovrd=off  show_param=off
      settings: xl_area=[0, 0, 0, 0, 0, 0, 0]
  Logical3 : xbsIndex_r3/Logical  logical_function=AND  inputs=2  precision=Full  arith_type=Unsigned  n_bits=8  bin_pt=2  align_bp=on  latency=0  explicit_period=off  period=1  en=off  dbl_ovrd=off  show_param=off
      settings: xl_area=[0, 0, 0, 0, 0, 0, 0]
  Logical4 : xbsIndex_r3/Logical  logical_function=OR  inputs=2  precision=Full  arith_type=Unsigned  n_bits=8  bin_pt=2  align_bp=off  latency=0  explicit_period=off  period=1  en=off  dbl_ovrd=off  show_param=off
      settings: xl_area=[0, 0, 0, 0, 0, 0, 0]
  Relational : xbsIndex_r3/Relational  mode=a>=b  latency=0  explicit_period=on  period=1  en=off  dbl_ovrd=off  show_param=off
      settings: xl_area=[0, 0, 0, 0, 0, 0, 0]
  Relational1 : xbsIndex_r3/Relational  mode=a=b  latency=0  explicit_period=on  period=1  en=off  dbl_ovrd=off  show_param=off
      settings: xl_area=[0, 0, 0, 0, 0, 0, 0]
  Relational2 : xbsIndex_r3/Relational  mode=a>b  latency=0  explicit_period=on  period=1  en=off  dbl_ovrd=off  show_param=off
      settings: xl_area=[0, 0, 0, 0, 0, 0, 0]
  Scope1 : Scope  NumInputPorts=4
      settings: YMin=0~-1~0~0  YMax=1~1~1~1
  Scope2 : Scope  NumInputPorts=4
      settings: YMin=0.95~0~-1~-5  YMax=1.05~1~1~5
  Slice6 : xbsIndex_r3/Slice  mode=Lower Bit Location + Width  nbits=1  bit1=3  base1=LSB of Input  bit0=0  base0=LSB of Input  boolean_output=on  explicit_period=off  period=1  dbl_ovrd=off
  edge1 : casper_library/Misc/edge
  group_cntr : xbsIndex_r3/Counter  cnt_type=Free Running  n_bits=32  bin_pt=0  arith_type=Unsigned  start_count=1  cnt_to=(floor(2^ant_bits / 2) + 1) * 2  cnt_by_val=1  operation=Up  explicit_period=on  period=1  load_pin=off  rst=on  en=off  dbl_ovrd=off  show_param=off  use_rpm=on  gen_core=off
      settings: xl_area=[0, 0, 0, 0, 0, 0, 0]
  posedge : casper_library/Misc/posedge  Tag=Rising Edge Detector
  pulse_cntr : xbsIndex_r3/Counter  cnt_type=Free Running  n_bits=32  bin_pt=0  arith_type=Unsigned  start_count=0  cnt_to=(floor(2^ant_bits / 2) + 1) * 2  cnt_by_val=1  operation=Up  explicit_period=on  period=1  load_pin=off  rst=on  en=on  dbl_ovrd=off  show_param=off  use_rpm=on  gen_core=off
      settings: xl_area=[0, 0, 0, 0, 0, 0, 0]
  tot_cntr : xbsIndex_r3/Counter  cnt_type=Free Running  n_bits=32  bin_pt=0  arith_type=Unsigned  start_count=1  cnt_to=(floor(2^ant_bits / 2) + 1) * 2  cnt_by_val=1  operation=Up  explicit_period=on  period=1  load_pin=off  rst=on  en=on  dbl_ovrd=off  show_param=off  use_rpm=on  gen_core=off
      settings: xl_area=[0, 0, 0, 0, 0, 0, 0]
  valid : Outport
  running : Outport  Port=2
  wires:
  tot_cntr/1 -> Relational/2, Gateway Out1/1
  Slice6/1 -> edge1/1
  run/1 -> posedge/1, Logical2/1, Gateway Out8/1
  Relational/1 -> running/1, Logical1/2, Gateway Out2/1, Logical2/3, Logical3/1
  num_pulses/1 -> Relational/1
  posedge/1 -> tot_cntr/1, Logical4/1, Gateway Out3/1
  group_cntr/1 -> Relational1/2, Gateway Out5/1
  Relational1/1 -> Logical4/2
  pulse_cntr/1 -> Relational2/2, Slice6/1, Gateway Out4/1
  Relational2/1 -> Logical2/2
  num_per_group/1 -> Relational2/1
  Logical2/1 -> pulse_cntr/2, Gateway Out7/1
  Logical4/1 -> group_cntr/1, pulse_cntr/1
  group period/1 -> Relational1/1
  Gateway Out5/1 -> Scope2/3
  Gateway Out4/1 -> Scope2/2
  Gateway Out6/1 -> Scope2/1
  Gateway Out1/1 -> Scope2/4
  Gateway Out7/1 -> Scope1/3
  Gateway Out3/1 -> Scope1/2
  Gateway Out8/1 -> Scope1/1
  Gateway Out2/1 -> Scope1/4
  edge1/1 -> Logical1/1, Logical3/2
  Logical1/1 -> valid/1, Gateway Out6/1
  Logical3/1 -> tot_cntr/2

== system test_dram_vacc_out/dram_tvg1/inject_vector ==
  new_acc_in : Inport  Port=1  LatchInput=off
  data_in : Inport  Port=2  LatchInput=off
  valid_in : Inport  Port=3  LatchInput=off
  vector : Inport  Port=4  LatchInput=off
  value : Inport  Port=5  LatchInput=off
  enable : Inport  Port=6  LatchInput=off
  Concat : xbsIndex_r3/Concat  num_inputs=2  explicit_period=off  period=1  dbl_ovrd=off
  Constant : xbsIndex_r3/Constant  const=0  equ=P=C  arith_type=Unsigned  n_bits=96  bin_pt=0  opselect=C  inp2=PCIN>>17  opr=+  inp1=P  carry=CIN  iostate=0  explicit_period=off  period=1  dbl_ovrd=off
  Delay : xbsIndex_r3/Delay  latency=2  reg_retiming=off  explicit_period=off  period=1  en=off  accept_only_valid=off  init_zero=on  dbl_ovrd=off  show_param=off
      settings: xl_area=[0, 0, 0, 0, 0, 0, 0]
  Delay1 : xbsIndex_r3/Delay  latency=2  reg_retiming=off  explicit_period=off  period=1  en=off  accept_only_valid=off  init_zero=on  dbl_ovrd=off  show_param=off
      settings: xl_area=[0, 0, 0, 0, 0, 0, 0]
  Delay2 : xbsIndex_r3/Delay  latency=2  reg_retiming=off  explicit_period=off  period=1  en=off  accept_only_valid=off  init_zero=on  dbl_ovrd=off  show_param=off
      settings: xl_area=[0, 0, 0, 0, 0, 0, 0]
  Delay3 : xbsIndex_r3/Delay  latency=3  reg_retiming=on  explicit_period=off  period=1  en=off  accept_only_valid=off  init_zero=on  dbl_ovrd=off  show_param=off
      settings: xl_area=[0, 0, 0, 0, 0, 0, 0]
  Delay4 : xbsIndex_r3/Delay  latency=1  reg_retiming=on  explicit_period=off  period=1  en=off  accept_only_valid=off  init_zero=on  dbl_ovrd=off  show_param=off
      settings: xl_area=[0, 0, 0, 0, 0, 0, 0]
  Gateway Out{1..2,4..6} (5 alike) : xbsIndex_r3/Gateway Out  output_type=Double  nbits=8  bin_pt=6  arith_type=Boolean  quantization=Truncate  overflow=Wrap  hdl_port=off  timing_constraint=None  locs_specified=off  LOCs={}  needs_fixed_name=off  show_param=off
      settings: xl_area=[0, 0, 0, 0, 0, 0, 0]
  Logical : xbsIndex_r3/Logical  logical_function=AND  inputs=2  precision=Full  arith_type=Unsigned  n_bits=8  bin_pt=2  align_bp=on  latency=0  explicit_period=off  period=1  en=off  dbl_ovrd=off  show_param=off
      settings: xl_area=[0, 0, 0, 0, 0, 0, 0]
  Mux : xbsIndex_r3/Mux  inputs=2  precision=Full  arith_type="Signed  (2's comp)"  n_bits=8  bin_pt=2  quantization=Truncate  overflow=Wrap  latency=1  explicit_period=off  period=1  en=off  dbl_ovrd=off  show_param=off  mux_type=off  use_rpm=off  gen_core=off
      settings: xl_area=[0, 0, 0, 0, 0, 0, 0]
  Relational : xbsIndex_r3/Relational  mode=a=b  latency=1  explicit_period=on  period=1  en=off  dbl_ovrd=off  show_param=off
      settings: xl_area=[0, 0, 0, 0, 0, 0, 0]
  Scope2 : Scope  NumInputPorts=5
      settings: YMin=0.95~0~-1~-5~-5  YMax=1.05~1~1~5~5
  posedge : casper_library/Misc/posedge  Tag=Rising Edge Detector
  tot_cntr : xbsIndex_r3/Counter  cnt_type=Count Limited  n_bits=32  bin_pt=0  arith_type=Unsigned  start_count=0  cnt_to=num_vectors-1  cnt_by_val=1  operation=Up  explicit_period=on  period=1  load_pin=off  rst=on  en=on  dbl_ovrd=off  show_param=off  use_rpm=on  gen_core=off
      settings: xl_area=[0, 0, 0, 0, 0, 0, 0]
  new_acc_out : Outport
  data : Outport  Port=2
  valid_out : Outport  Port=3
  wires:
  enable/1 -> Logical/1
  posedge/1 -> tot_cntr/1, Gateway Out1/1
  Gateway Out5/1 -> Scope2/3
  Gateway Out4/1 -> Scope2/2
  Gateway Out6/1 -> Scope2/1
  Gateway Out1/1 -> Scope2/4
  valid_in/1 -> Delay4/1
  Mux/1 -> data/1, Gateway Out6/1
  tot_cntr/1 -> Gateway Out2/1, Relational/1
  vector/1 -> Relational/2
  data_in/1 -> Delay1/1
  value/1 -> Delay2/1
  Delay/1 -> valid_out/1, Gateway Out4/1
  Logical/1 -> Mux/1
  Relational/1 -> Logical/2
  Gateway Out2/1 -> Scope2/5
  Delay1/1 -> Mux/2
  Delay3/1 -> new_acc_out/1
  new_acc_in/1 -> Delay3/1, posedge/1
  Delay4/1 -> tot_cntr/2, Delay/1, Gateway Out5/1
  Delay2/1 -> Concat/2
  Concat/1 -> Mux/3
  Constant/1 -> Concat/1

== system test_dram_vacc_out/dram_tvg1/insert_counter ==
  new_acc_in : Inport  Port=1  LatchInput=off
  din : Inport  Port=2  LatchInput=off
  valid_in : Inport  Port=3  LatchInput=off
  enable : Inport  Port=4  LatchInput=off
  Concat : xbsIndex_r3/Concat  num_inputs=2  explicit_period=off  period=1  dbl_ovrd=off
  Counter : xbsIndex_r3/Counter  cnt_type=Count Limited  n_bits=32  bin_pt=0  arith_type=Unsigned  start_count=0  cnt_to=vec_len-1  cnt_by_val=1  operation=Up  explicit_period=off  period=1  load_pin=off  rst=on  en=on  dbl_ovrd=off  show_param=off  use_rpm=on  gen_core=off
      settings: xl_area=[0, 0, 0, 0, 0, 0, 0]
  Delay{,1..3} (4 alike) : xbsIndex_r3/Delay  latency=1  reg_retiming=on  explicit_period=off  period=1  en=off  accept_only_valid=off  init_zero=on  dbl_ovrd=off  show_param=off
      settings: xl_area=[0, 0, 0, 0, 0, 0, 0]
  Gateway Out4 : xbsIndex_r3/Gateway Out  output_type=Double  nbits=8  bin_pt=6  arith_type=Boolean  quantization=Truncate  overflow=Wrap  hdl_port=off  timing_constraint=None  locs_specified=off  LOCs={}  needs_fixed_name=off  show_param=off
      settings: xl_area=[0, 0, 0, 0, 0, 0, 0]
  Gateway Out5 : xbsIndex_r3/Gateway Out  output_type=Double  nbits=8  bin_pt=6  arith_type=Boolean  quantization=Truncate  overflow=Wrap  hdl_port=off  timing_constraint=None  locs_specified=off  LOCs={}  needs_fixed_name=off  show_param=off
      settings: xl_area=[0, 0, 0, 0, 0, 0, 0]
  Gateway Out6 : xbsIndex_r3/Gateway Out  output_type=Double  nbits=8  bin_pt=6  arith_type=Boolean  quantization=Truncate  overflow=Wrap  hdl_port=off  timing_constraint=None  locs_specified=off  LOCs={}  needs_fixed_name=off  show_param=off
      settings: xl_area=[0, 0, 0, 0, 0, 0, 0]
  Mux : xbsIndex_r3/Mux  inputs=2  precision=Full  arith_type="Signed  (2's comp)"  n_bits=8  bin_pt=2  quantization=Truncate  overflow=Wrap  latency=0  explicit_period=off  period=1  en=off  dbl_ovrd=off  show_param=off  mux_type=off  use_rpm=off  gen_core=off
      settings: xl_area=[0, 0, 0, 0, 0, 0, 0]
  Scope2 : Scope  NumInputPorts=3
      settings: YMin=-1~65~0  YMax=1~92.5~1  SaveName=ScopeData35
  Slice2 : xbsIndex_r3/Slice  mode=Lower Bit Location + Width  nbits=32  bit1=3  base1=LSB of Input  bit0=0  base0=LSB of Input  boolean_output=off  explicit_period=on  period=1  dbl_ovrd=off
  Slice3 : xbsIndex_r3/Slice  mode=Upper Bit Location + Width  nbits=96  bit1=0  base1=MSB of Input  bit0=0  base0=LSB of Input  boolean_output=off  explicit_period=on  period=1  dbl_ovrd=off
  posedge : casper_library/Misc/posedge  Tag=Rising Edge Detector
  new_acc_out : Outport
  dout : Outport  Port=2
  valid_out : Outport  Port=3
  wires:
  new_acc_in/1 -> Delay/1, posedge/1
  valid_in/1 -> Delay1/1, Delay3/1
  enable/1 -> Mux/1
  din/1 -> Delay2/1
  Slice2/1 -> Mux/2
  Counter/1 -> Mux/3, Gateway Out4/1
  Slice3/1 -> Concat/1
  Mux/1 -> Concat/2
  Concat/1 -> dout/1
  Delay/1 -> new_acc_out/1
  Delay1/1 -> valid_out/1
  Delay2/1 -> Slice2/1, Slice3/1
  posedge/1 -> Counter/1, Gateway Out6/1
  Gateway Out5/1 -> Scope2/3
  Gateway Out4/1 -> Scope2/2
  Gateway Out6/1 -> Scope2/1
  Delay3/1 -> Counter/2, Gateway Out5/1
